simulink model "Ext_Light"  (R2020b)
settings: Solver=VariableStepAuto  StartTime=0.0  StopTime=10.0  RelTol=1e-3
settings Model: Creator=sharath chandra  LastModifiedBy=sharath chandra

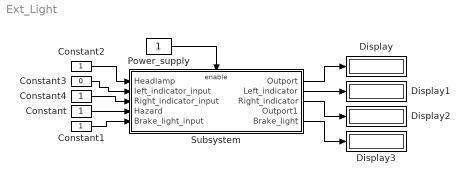
== system Ext_Light ==
  Constant{,1..2,4} (4 alike) : Constant
  Constant3 : Constant  Value=0
  Display{,1..3} (4 alike) : Display
  Power_supply : Constant
  Subsystem : Subsystem
  wires:
  Constant/1 -> Subsystem/4(Hazard)
  Constant1/1 -> Subsystem/5(Brake_light_input)
  Constant2/1 -> Subsystem/1(Headlamp)
  Constant3/1 -> Subsystem/2(Ieft_indicator_input)
  Constant4/1 -> Subsystem/3(Right_indicator_input)
  Subsystem/1(Outport) -> Display/1
  Subsystem/2(Left_indicator) -> Display1/1
  Subsystem/3(Right_indicator) -> Display2/1
  Subsystem/5(Brake_light) -> Display3/1
  Power_supply/1 -> Subsystem/Enable

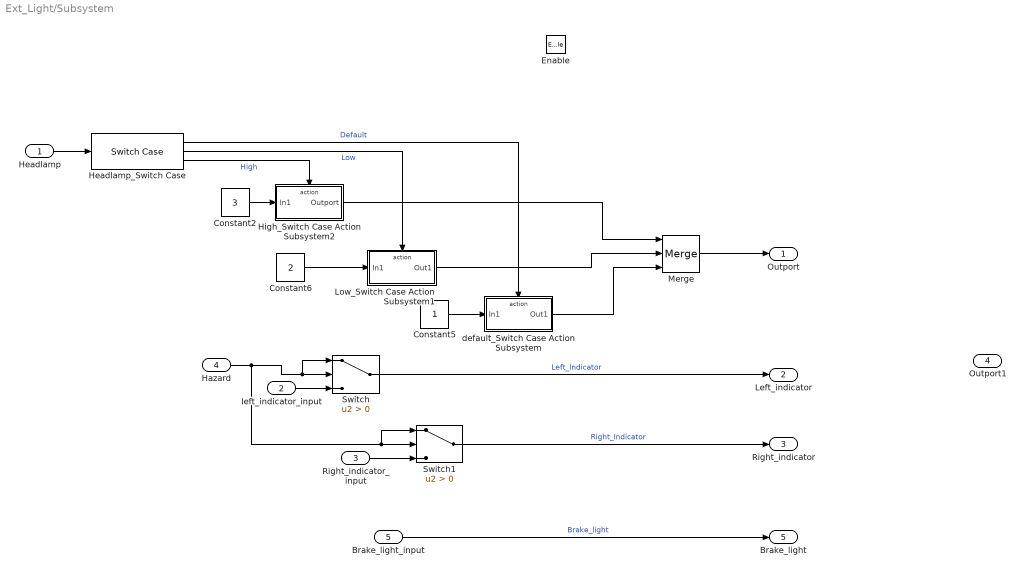
== system Ext_Light/Subsystem ==
  Headlamp : Inport
  Ieft_indicator_input : Inport  Port=2
  Right_indicator_input : Inport  Port=3
  Hazard : Inport  Port=4
  Brake_light_input : Inport  Port=5
  Enable : EnablePort
  Constant2 : Constant  Value=3
  Constant5 : Constant
  Constant6 : Constant  Value=2
  Headlamp_Switch Case : SwitchCase  CaseConditions={0,-1,1}  ShowDefaultCase=off
  High_Switch Case Action Subsystem2 : Subsystem  TreatAsAtomicUnit=on
  Low_Switch Case Action Subsystem1 : Subsystem  TreatAsAtomicUnit=on
  Merge : Merge  Inputs=3
  Switch : Switch  Criteria=u2 > Threshold
  Switch1 : Switch  Criteria=u2 > Threshold
  default_Switch Case Action Subsystem : Subsystem  TreatAsAtomicUnit=on
  Outport : Outport
  Left_indicator : Outport  Port=2
  Right_indicator : Outport  Port=3
  Outport1 : Outport  Port=4
  Brake_light : Outport  Port=5
  wires:
  Constant5/1 -> default_Switch Case Action Subsystem/1(In1)
  Headlamp_Switch Case/2 -> Low_Switch Case Action Subsystem1/Action  "Low"
  High_Switch Case Action Subsystem2/1(Outport) -> Merge/1
  Merge/1 -> Outport/1
  Constant2/1 -> High_Switch Case Action Subsystem2/1(In1)
  Headlamp_Switch Case/1 -> default_Switch Case Action Subsystem/Action  "Default"
  Headlamp_Switch Case/3 -> High_Switch Case Action Subsystem2/Action  "High"
  default_Switch Case Action Subsystem/1(Out1) -> Merge/3
  Headlamp/1 -> Headlamp_Switch Case/1
  Constant6/1 -> Low_Switch Case Action Subsystem1/1(In1)
  Low_Switch Case Action Subsystem1/1(Out1) -> Merge/2
  Ieft_indicator_input/1 -> Switch/3
  Switch/1 -> Left_indicator/1  "Left_Indicator"
  Hazard/1 -> Switch1/1, Switch1/2, Switch/1, Switch/2
  Right_indicator_input/1 -> Switch1/3
  Switch1/1 -> Right_indicator/1  "Right_Indicator"
  Brake_light_input/1 -> Brake_light/1  "Brake_light"

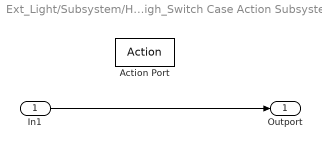
== system Ext_Light/Subsystem/High_Switch Case Action Subsystem2 ==
  In1 : Inport
  Action Port : ActionPort  ActionPortLabel=case [ 1 ]:
  Outport : Outport
  wires:
  In1/1 -> Outport/1

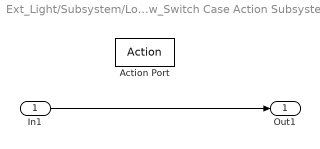
== system Ext_Light/Subsystem/Low_Switch Case Action Subsystem1 ==
  In1 : Inport
  Action Port : ActionPort  ActionPortLabel=case [ -1 ]:
  Out1 : Outport
  wires:
  In1/1 -> Out1/1

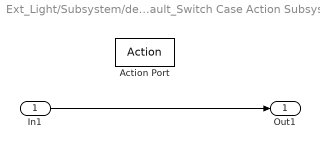
== system Ext_Light/Subsystem/default_Switch Case Action Subsystem ==
  In1 : Inport
  Action Port : ActionPort  ActionPortLabel=case [ 0 ]:
  Out1 : Outport
  wires:
  In1/1 -> Out1/1
